simulink model "eVTOL"  (R2021b)
settings: Solver=VariableStepAuto  StartTime=0.0  StopTime=60  RelTol=1e-3
settings Model: Creator=ywu86  LastModifiedBy=ywu86

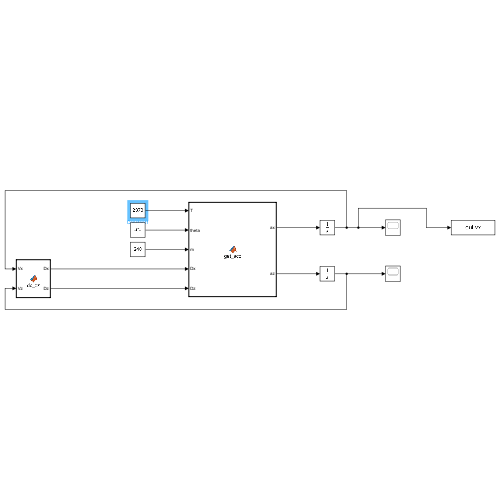
[thumbnail: Simulink's stored preview of the top-level diagram]
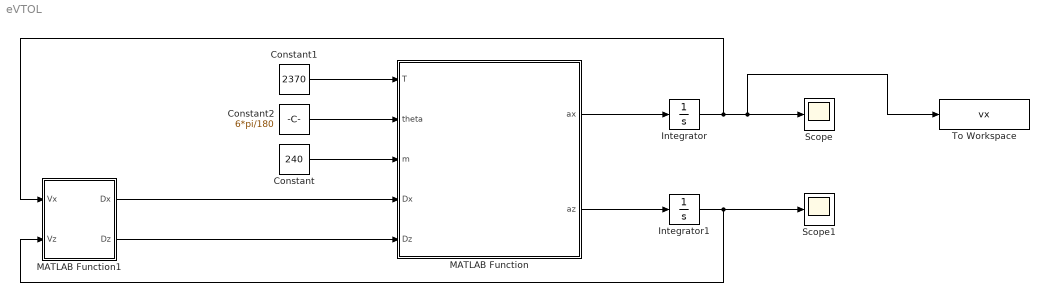
== system eVTOL ==
  Constant : Constant  Value=240
  Constant1 : Constant  Value=2370
  Constant2 : Constant  Value=6*pi/180
  Integrator : Integrator
  Integrator1 : Integrator
  MATLAB Function : MATLAB Function  TreatAsAtomicUnit=on
  MATLAB Function1 : MATLAB Function  TreatAsAtomicUnit=on
  Scope : Scope
  Scope1 : Scope
  To Workspace : ToWorkspace  VariableName=vx  SaveFormat=Timeseries  SampleTime=0.1
  wires:
  MATLAB Function1/1(Dx) -> MATLAB Function/4(Dx)
  MATLAB Function1/2(Dz) -> MATLAB Function/5(Dz)
  Constant/1 -> MATLAB Function/3(m)
  Constant2/1 -> MATLAB Function/2(theta)
  Constant1/1 -> MATLAB Function/1(T)
  MATLAB Function/1(ax) -> Integrator/1
  MATLAB Function/2(az) -> Integrator1/1
  Integrator1/1 -> Scope1/1, MATLAB Function1/2(Vz)
  Integrator/1 -> To Workspace/1, Scope/1, MATLAB Function1/1(Vx)

== matlab function eVTOL/MATLAB Function1 ==
  data: Vx input; Dx output; Vz input; Dz output
function [Dx, Dz] = dx_dz(Vx,Vz)
pho = 1.225;
m=240;
Sx     = 2.11;          % vehicle's frontal area, m^2
Sz     = 1.47;          % drag coefficient
g      = 9.81;          % gravitaional acceleration, m/s^2
CD     = 1;             % drag coefficient
Dx = (pho*Vx^2*CD*Sx)/2;
Dz = (pho*Vz^2*CD*Sz)/2;

== matlab function eVTOL/MATLAB Function ==
  data: T input; ax output; theta input; m input; Dx input; Dz input; az output
function [ax,az] = get_acc(T,theta,m,Dx,Dz)
    ax = (T*sin(theta)/m)-Dx/m;
    az = (T*cos(theta)/m)-Dz/m-9.81;
